simulink model "nnn_cassie_sims"  (R2017b)
settings: Solver=VariableStepAuto  StartTime=0.0  StopTime=30
InitFcn:
  | PreFunctionss.PreParamss;
  | PreFunctionss.GaitData;
model workspace (MATLAB code in the model file):
  | PreFunctionss.BusInfoss
  | PreFunctionss.BusDataS
values from neighbouring files (symbols this model uses):
  s = min(s_unsat,1.05)    [ControllerS.m]
undefined symbols (not defined in the file or in its folder): fcut_velocity_joint, GaitLibrary, motorPositions, motorVelocities, pelvisPosition, pelvisVelocity, sampleTime, X, Y, Z
libraries: sm_lib x83, nesl_utility x17, ComponentLibrary x10, Contact_Forces_Lib x4, CassieLibrary x4, etargetslib x1, instrumentlib x1, simulink x1
(part 4 of 4)

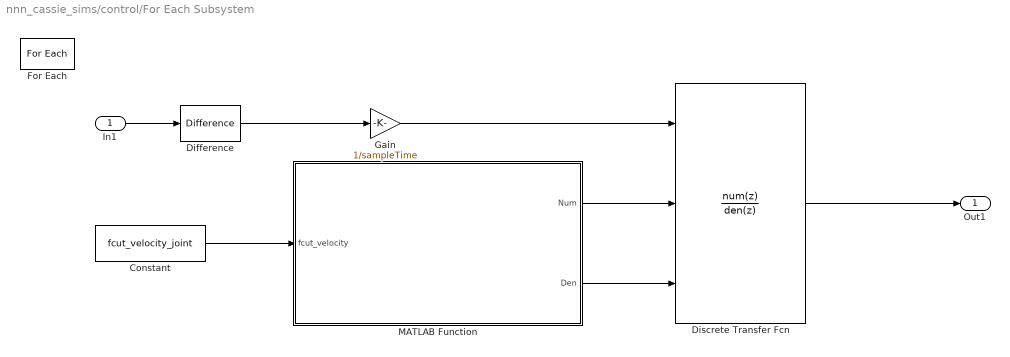
== system nnn_cassie_sims/control/For Each Subsystem ==
  In1 : Inport  Partition=on  PartitionDimension=1  PartitionWidth=1  PartitionOffset=0
  Constant : Constant  Value=fcut_velocity_joint
  Difference : simulink/Discrete/Difference  ICPrevInput=0.0  OutMin=[]  OutMax=[]  OutDataType=fixdt(1, 16)  OutScaling=2^-10  DoSatur=off
  Discrete Transfer Fcn : DiscreteTransferFcn  NumeratorSource=Input port  DenominatorSource=Input port  SampleTime=sampleTime  a0EqualsOne=on
      settings: InputPortMap=u0,p1,p3
  For Each : ForEach  DisableCoverage=on  IndexMode=One-based
  Gain : Gain  Gain=1/sampleTime
  MATLAB Function : MATLAB Function  TreatAsAtomicUnit=on
  Out1 : Outport  ConcatenationDimension=1
  wires:
  In1/1 -> Difference/1
  Difference/1 -> Gain/1
  Constant/1 -> MATLAB Function/1(fcut_velocity)
  Discrete Transfer Fcn/1 -> Out1/1
  Gain/1 -> Discrete Transfer Fcn/1
  MATLAB Function/1(Num) -> Discrete Transfer Fcn/2
  MATLAB Function/2(Den) -> Discrete Transfer Fcn/3

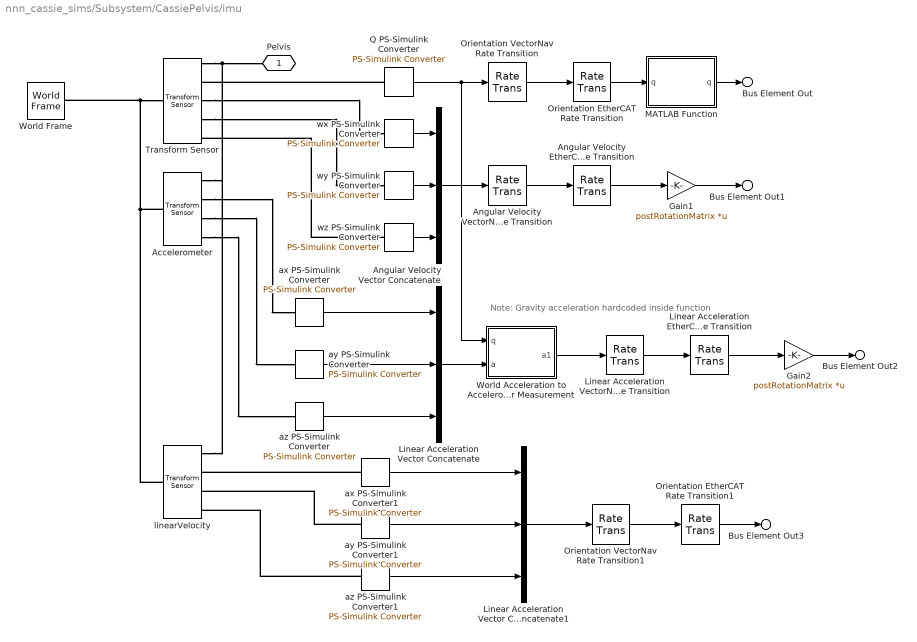
== system nnn_cassie_sims/Subsystem/CassiePelvis/imu ==
  note: Note: Gravity acceleration hardcoded inside function
  Accelerometer : sm_lib/Frames and Transforms/Transform Sensor  MeasurementFrame=Base  SenseAngle=off  SenseAxis=off  SenseAngle1=off  SenseAngle2=off  SenseAngle3=off  SenseQ=off  SenseR=off  SenseOmegaX=off  SenseOmegaY=off  SenseOmegaZ=off  SenseOmega1=off  SenseOmega2=off  SenseOmega3=off  SenseQDot=off  SenseRDot=off  SenseAlphaX=off  SenseAlphaY=off  SenseAlphaZ=off  SenseAlpha1=off  SenseAlpha2=off  SenseAlpha3=off  SenseQDDot=off  SenseRDDot=off  SenseX=off  SenseY=off  SenseZ=off  SenseRad=off  SenseAzim=off  SenseDist=off  SenseInc=off  SenseXDot=off  SenseYDot=off  SenseZDot=off  SenseRadDot=off  SenseAzimDot=off  SenseDistDot=off  SenseIncDot=off  SenseXDDot=on  SenseYDDot=on  SenseZDDot=on  SenseRadDDot=off  SenseAzimDDot=off  SenseDistDDot=off  SenseIncDDot=off
  Angular Velocity EtherCAT Rate Transition : RateTransition  Deterministic=off  OutPortSampleTimeOpt=Inherit
  Angular Velocity Vector Concatenate : Concatenate  NumInputs=3
  Angular Velocity VectorNav Rate Transition : RateTransition  Deterministic=off  OutPortSampleTime=sampleTime
  Gain1 : Gain  Gain=postRotationMatrix  Multiplication=Matrix(K*u)
  Gain2 : Gain  Gain=postRotationMatrix  Multiplication=Matrix(K*u)
  Linear Acceleration EtherCAT Rate Transition : RateTransition  Deterministic=off  InitialCondition=[0; 0; 0]  OutPortSampleTimeOpt=Inherit
  Linear Acceleration Vector Concatenate : Concatenate  NumInputs=3
  Linear Acceleration Vector Concatenate1 : Concatenate  NumInputs=3
  Linear Acceleration VectorNav Rate Transition : RateTransition  Deterministic=off  InitialCondition=[0; 0; 0]  OutPortSampleTime=sampleTime
  MATLAB Function : MATLAB Function  TreatAsAtomicUnit=on
  Orientation EtherCAT Rate Transition : RateTransition  Deterministic=off  InitialCondition=[0; 0; 0; 1]  OutPortSampleTimeOpt=Inherit
  Orientation EtherCAT Rate Transition1 : RateTransition  Deterministic=off  InitialCondition=[0; 0; 0]  OutPortSampleTimeOpt=Inherit
  Orientation VectorNav Rate Transition : RateTransition  Deterministic=off  InitialCondition=[0; 0; 0; 1]  OutPortSampleTime=sampleTime
  Orientation VectorNav Rate Transition1 : RateTransition  Deterministic=off  InitialCondition=[0; 0; 0]  OutPortSampleTime=sampleTime
  Q PS-Simulink Converter : nesl_utility/PS-Simulink Converter  PhysicalDomain=network_engine_domain  SubClassName=ps_output  LeftPortType=input  RightPortType=output  PseudoPeriodic=off  Frequencies=[]  Unit=1  AffineConversion=off
  Transform Sensor : sm_lib/Frames and Transforms/Transform Sensor  MeasurementFrame=Follower  SenseAngle=off  SenseAxis=off  SenseAngle1=off  SenseAngle2=off  SenseAngle3=off  SenseQ=on  SenseR=off  SenseOmegaX=on  SenseOmegaY=on  SenseOmegaZ=on  SenseOmega1=off  SenseOmega2=off  SenseOmega3=off  SenseQDot=off  SenseRDot=off  SenseAlphaX=off  SenseAlphaY=off  SenseAlphaZ=off  SenseAlpha1=off  SenseAlpha2=off  SenseAlpha3=off  SenseQDDot=off  SenseRDDot=off  SenseX=off  SenseY=off  SenseZ=off  SenseRad=off  SenseAzim=off  SenseDist=off  SenseInc=off  SenseXDot=off  SenseYDot=off  SenseZDot=off  SenseRadDot=off  SenseAzimDot=off  SenseDistDot=off  SenseIncDot=off  SenseXDDot=off  SenseYDDot=off  SenseZDDot=off  SenseRadDDot=off  SenseAzimDDot=off  SenseDistDDot=off  SenseIncDDot=off
  World Acceleration to Accelerometer Measurement : MATLAB Function  TreatAsAtomicUnit=on
  World Frame : sm_lib/Frames and Transforms/World Frame
  ax PS-Simulink Converter : nesl_utility/PS-Simulink Converter  PhysicalDomain=network_engine_domain  SubClassName=ps_output  LeftPortType=input  RightPortType=output  PseudoPeriodic=off  Frequencies=[]  Unit=m/s/s  AffineConversion=off
  ax PS-Simulink Converter1 : nesl_utility/PS-Simulink Converter  PhysicalDomain=network_engine_domain  SubClassName=ps_output  LeftPortType=input  RightPortType=output  PseudoPeriodic=off  Frequencies=[]  Unit=m/s  AffineConversion=off
  ay PS-Simulink Converter : nesl_utility/PS-Simulink Converter  PhysicalDomain=network_engine_domain  SubClassName=ps_output  LeftPortType=input  RightPortType=output  PseudoPeriodic=off  Frequencies=[]  Unit=m/s/s  AffineConversion=off
  ay PS-Simulink Converter1 : nesl_utility/PS-Simulink Converter  PhysicalDomain=network_engine_domain  SubClassName=ps_output  LeftPortType=input  RightPortType=output  PseudoPeriodic=off  Frequencies=[]  Unit=m/s  AffineConversion=off
  az PS-Simulink Converter : nesl_utility/PS-Simulink Converter  PhysicalDomain=network_engine_domain  SubClassName=ps_output  LeftPortType=input  RightPortType=output  PseudoPeriodic=off  Frequencies=[]  Unit=m/s/s  AffineConversion=off
  az PS-Simulink Converter1 : nesl_utility/PS-Simulink Converter  PhysicalDomain=network_engine_domain  SubClassName=ps_output  LeftPortType=input  RightPortType=output  PseudoPeriodic=off  Frequencies=[]  Unit=m/s  AffineConversion=off
  linearVelocity : sm_lib/Frames and Transforms/Transform Sensor  MeasurementFrame=Base  SenseAngle=off  SenseAxis=off  SenseAngle1=off  SenseAngle2=off  SenseAngle3=off  SenseQ=off  SenseR=off  SenseOmegaX=off  SenseOmegaY=off  SenseOmegaZ=off  SenseOmega1=off  SenseOmega2=off  SenseOmega3=off  SenseQDot=off  SenseRDot=off  SenseAlphaX=off  SenseAlphaY=off  SenseAlphaZ=off  SenseAlpha1=off  SenseAlpha2=off  SenseAlpha3=off  SenseQDDot=off  SenseRDDot=off  SenseX=off  SenseY=off  SenseZ=off  SenseRad=off  SenseAzim=off  SenseDist=off  SenseInc=off  SenseXDot=on  SenseYDot=on  SenseZDot=on  SenseRadDot=off  SenseAzimDot=off  SenseDistDot=off  SenseIncDot=off  SenseXDDot=off  SenseYDDot=off  SenseZDDot=off  SenseRadDDot=off  SenseAzimDDot=off  SenseDistDDot=off  SenseIncDDot=off
  wx PS-Simulink Converter : nesl_utility/PS-Simulink Converter  PhysicalDomain=network_engine_domain  SubClassName=ps_output  LeftPortType=input  RightPortType=output  PseudoPeriodic=off  Frequencies=[]  Unit=1  AffineConversion=off
  wy PS-Simulink Converter : nesl_utility/PS-Simulink Converter  PhysicalDomain=network_engine_domain  SubClassName=ps_output  LeftPortType=input  RightPortType=output  PseudoPeriodic=off  Frequencies=[]  Unit=1  AffineConversion=off
  wz PS-Simulink Converter : nesl_utility/PS-Simulink Converter  PhysicalDomain=network_engine_domain  SubClassName=ps_output  LeftPortType=input  RightPortType=output  PseudoPeriodic=off  Frequencies=[]  Unit=1  AffineConversion=off
  Pelvis : PMIOPort  Port=1  Side=Left
  Bus Element Out1 : Outport  PortName=OutBus  Element=angularVelocity
  Bus Element Out2 : Outport  PortName=OutBus  Element=linearAcceleration
  Bus Element Out : Outport  PortName=OutBus  Element=orientation
  Bus Element Out3 : Outport  PortName=OutBus  Element=linearVelocity
  wires:
  Angular Velocity VectorNav Rate Transition/1 -> Angular Velocity EtherCAT Rate Transition/1
  wz PS-Simulink Converter/1 -> Angular Velocity Vector Concatenate/3
  wx PS-Simulink Converter/1 -> Angular Velocity Vector Concatenate/1
  Orientation EtherCAT Rate Transition/1 -> MATLAB Function/1("q ")
  Q PS-Simulink Converter/1 -> World Acceleration to Accelerometer Measurement/1(q), Orientation VectorNav Rate Transition/1
  wy PS-Simulink Converter/1 -> Angular Velocity Vector Concatenate/2
  Angular Velocity EtherCAT Rate Transition/1 -> Gain1/1
  Orientation VectorNav Rate Transition/1 -> Orientation EtherCAT Rate Transition/1
  Linear Acceleration EtherCAT Rate Transition/1 -> Gain2/1
  Linear Acceleration VectorNav Rate Transition/1 -> Linear Acceleration EtherCAT Rate Transition/1
  Angular Velocity Vector Concatenate/1 -> Angular Velocity VectorNav Rate Transition/1
  Gain1/1 -> Bus Element Out1/1
  MATLAB Function/1(q) -> Bus Element Out/1
  ax PS-Simulink Converter/1 -> Linear Acceleration Vector Concatenate/1
  ay PS-Simulink Converter/1 -> Linear Acceleration Vector Concatenate/2
  az PS-Simulink Converter/1 -> Linear Acceleration Vector Concatenate/3
  Gain2/1 -> Bus Element Out2/1
  World Acceleration to Accelerometer Measurement/1(a1) -> Linear Acceleration VectorNav Rate Transition/1
  Linear Acceleration Vector Concatenate/1 -> World Acceleration to Accelerometer Measurement/2(a)
  az PS-Simulink Converter1/1 -> Linear Acceleration Vector Concatenate1/3
  ay PS-Simulink Converter1/1 -> Linear Acceleration Vector Concatenate1/2
  ax PS-Simulink Converter1/1 -> Linear Acceleration Vector Concatenate1/1
  Orientation VectorNav Rate Transition1/1 -> Orientation EtherCAT Rate Transition1/1
  Linear Acceleration Vector Concatenate1/1 -> Orientation VectorNav Rate Transition1/1
  Orientation EtherCAT Rate Transition1/1 -> Bus Element Out3/1
  connections:
  Transform Sensor/RConn4 -- wy PS-Simulink Converter/LConn1
  Accelerometer/LConn1 -- linearVelocity/LConn1 -- World Frame/RConn1 -- Transform Sensor/LConn1
  Accelerometer/RConn3 -- ay PS-Simulink Converter/LConn1
  Q PS-Simulink Converter/LConn1 -- Transform Sensor/RConn2
  Accelerometer/RConn2 -- ax PS-Simulink Converter/LConn1
  Transform Sensor/RConn1 -- linearVelocity/RConn1 -- Accelerometer/RConn1 -- Pelvis/RConn1
  Accelerometer/RConn4 -- az PS-Simulink Converter/LConn1
  Transform Sensor/RConn3 -- wx PS-Simulink Converter/LConn1
  wz PS-Simulink Converter/LConn1 -- Transform Sensor/RConn5
  ay PS-Simulink Converter1/LConn1 -- linearVelocity/RConn3
  az PS-Simulink Converter1/LConn1 -- linearVelocity/RConn4
  ax PS-Simulink Converter1/LConn1 -- linearVelocity/RConn2

== matlab function nnn_cassie_sims/Subsystem/CassiePelvis/imu/MATLAB Function ==
  data: q input; q output; preRotationMatrix parameter; postRotationMatrix parameter
function q = fcn(q, preRotationMatrix, postRotationMatrix)
  % Construct constant rotation matrix objects
  R0 = coder.const(Rotation3d(preRotationMatrix));
  R2 = coder.const(Rotation3d(postRotationMatrix));
  
  % Convert rotation matrices into constant quaternion objects
  Q0 = coder.const(R0.getQuaternion);
  Q2 = coder.const(R2.getQuaternion);
  
  % Apply pre and post rotations
  Q1 = Q0*Quaternion(q)*Q2;
  
  % Convert quaternion object to double
  q = Q1.getValue;
end % fcn

== matlab function nnn_cassie_sims/Subsystem/CassiePelvis/imu/World Acceleration to Accelerometer Measurement ==
  data: q input; a1 output; a input
function a1 = fcn(q, a)
  % Construct quaternion object
  Q = Quaternion(q);
  
  % Add world gravity acceleration to body acceleration
  a1 = Q.getRotation.getValue'*(a + [0; 0; -9.806]);
end % fcn

== matlab function nnn_cassie_sims/control/For Each Subsystem/MATLAB Function ==
  data: fcut_velocity input; Num output; Den output
function [Num, Den] = velocity_filter_param(fcut_velocity)
sample_time = 1/2000;
lpf_damping = sqrt(2)/2; % Butterworth filter damping
B1_lpf_velocity = -2*exp(-lpf_damping*fcut_velocity*sample_time)*cos(fcut_velocity*sample_time*sqrt(1-lpf_damping^2));
B2_lpf_velocity = exp(-2*lpf_damping*fcut_velocity*sample_time);
A_lpf_velocity = 1 + B1_lpf_velocity + B2_lpf_velocity;

Num = [ A_lpf_velocity 0 0];
Den = [ 1 B1_lpf_velocity B2_lpf_velocity];
end
